simulink model "district_screening"  (R2026a)
settings: Solver=VariableStepDiscrete  StopTime=120000
PreLoadFcn:
  | assignin('base', 'PatientBus', districtBus());
InitFcn:
  | assignin('base', 'PatientBus', districtBus());
model workspace (MAT data in the model file):
  params.annualPatients = 100000
  params.workingDays = 250
  params.referablePrevalence = 0.06
  params.anyDrPrevalence = 0.18
  params.phcs = 30
  params.camerasPerPhc = 1
  params.operatorsPerPhc = 1
  params.captureMinutes = 4
  params.retakeProbability = 0.002
  params.phcHoursPerDay = 8
  params.aiEnabled = 1
  params.sensitivity = 0.9467
  params.specificity = 0.8888
  params.flagRate = 0.2515
  params.humanReaderSensitivity = 0.85
  params.humanReaderSpecificity = 0.9
  params.ophthalmologists = 2
  params.doctorHoursPerDay = 6
  params.teleReviewMinutes = 3
  params.inPersonMinutes = 20
  params.operatorHourCost = 150
  params.doctorHourCost = 1500
  params.cameraAnnualCost = 50000
  params.seed = 42
  params.sampleFraction = 1
undefined symbols (not defined in the file or in its folder): m
settings Model: Creator=anilm  LastModifiedBy=anilm

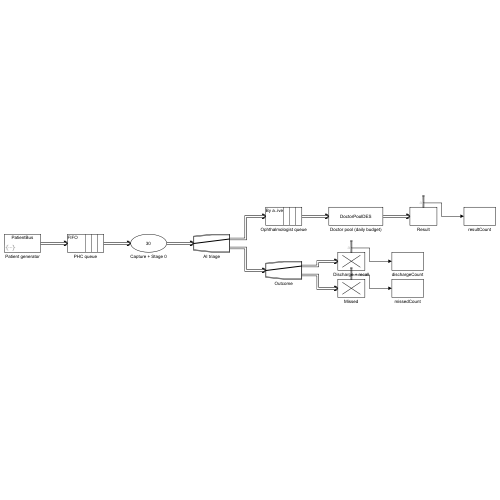
[thumbnail: Simulink's stored preview of the top-level diagram]
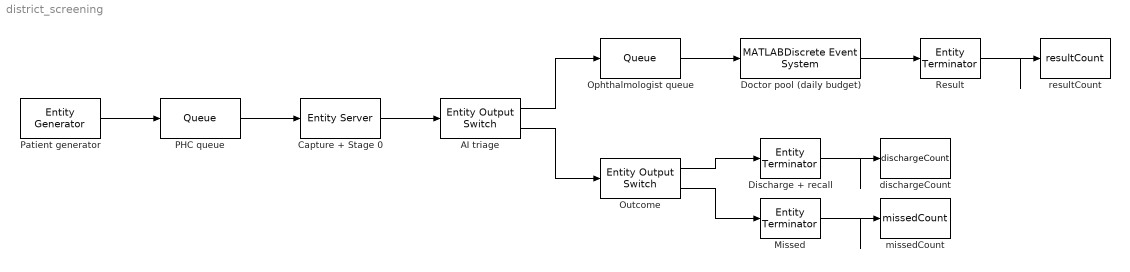
== system district_screening ==
  AI triage : EntityOutputSwitch  InputPortMessageModes=m  OutputPortMessageModes=m,m  SwitchingCriterion=From attribute  SwitchAttributeName=route
  Capture + Stage 0 : EntityServer  InputPortMessageModes=m  OutputPortMessageModes=m  Capacity=30  ServiceTimeSource=Attribute  ServiceTimeAttributeName=captureMinutes
  Discharge + recall : EntityTerminator  InputPortMessageModes=m  NumberEntitiesArrived=on
      settings: OutputPortMap=o0
  Doctor pool (daily budget) : MATLABDiscreteEventSystem  InputPortMessageModes=m  OutputPortMessageModes=m  System=DoctorPoolDES  NumDoctors=params.ophthalmologists  DailyBudgetMinutes=params.doctorHoursPerDay * 60  DayMinutes=params.phcHoursPerDay * 60  SimulateUsing=Code generation
      mask Type: DoctorPoolDES
  Missed : EntityTerminator  InputPortMessageModes=m  NumberEntitiesArrived=on
      settings: OutputPortMap=o0
  Ophthalmologist queue : Queue  InputPortMessageModes=m  OutputPortMessageModes=m  Capacity=inf  QueueType=Priority  PrioritySource=aiPositive  SortingDirection=Descending
  Outcome : EntityOutputSwitch  InputPortMessageModes=m  OutputPortMessageModes=m,m  SwitchingCriterion=From attribute  SwitchAttributeName=outcome
  PHC queue : Queue  InputPortMessageModes=m  OutputPortMessageModes=m  Capacity=inf
  Patient generator : EntityGenerator  OutputPortMessageModes=m  TimeSource=MATLAB action  IntergenerationTimeAction=dt = -1.2 * log(rand);  GenerateAction=|  EntityType=Bus object  EntityTypeName=PatientBus
      | entity.referable = double(rand < 0.06);
      | if entity.referable, entity.aiPositive = double(rand < 0.9467); else, entity.aiPositive = double(rand < 0.1112); end
      | entity.flagged = double(rand < 0.2515);
      | entity.toDoctor = double(1 && (entity.aiPositive || entity.flagged)) + double(~1);
      | entity.route = 2 - entity.toDoctor;
      | if entity.referable, entity.readerCalls = double(rand < 0.85); else, entity.readerCalls = double(rand < 0.1); end
      | entity.captureMinutes = 4 * (1 + double(rand < 0.002));
      | entity.reviewMinutes = 3 + 20 * entity.readerCalls;
      | entity.outcome = 1 + entity.referable;
  Result : EntityTerminator  InputPortMessageModes=m  NumberEntitiesArrived=on
      settings: OutputPortMap=o0
  dischargeCount : ToWorkspace  VariableName=dischargeCount  SaveFormat=Timeseries  SampleTime=-1
  missedCount : ToWorkspace  VariableName=missedCount  SaveFormat=Timeseries  SampleTime=-1
  resultCount : ToWorkspace  VariableName=resultCount  SaveFormat=Timeseries  SampleTime=-1
  wires:
  Patient generator/1 -> PHC queue/1
  PHC queue/1 -> Capture + Stage 0/1
  Capture + Stage 0/1 -> AI triage/1
  AI triage/2 -> Outcome/1
  Outcome/1 -> Discharge + recall/1
  Outcome/2 -> Missed/1
  Doctor pool (daily budget)/1 -> Result/1
  AI triage/1 -> Ophthalmologist queue/1
  Ophthalmologist queue/1 -> Doctor pool (daily budget)/1
  Result/1 -> resultCount/1
  Discharge + recall/1 -> dischargeCount/1
  Missed/1 -> missedCount/1
